simulink model "zad73_dir2slx"  (R2015a)
settings: Solver=FixedStepDiscrete  StartTime=0.0  StopTime=99.0  FixedStep=1  RelTol=1e-3
settings Model: Creator=Bojana Vasic  LastModifiedBy=Bojana Vasic

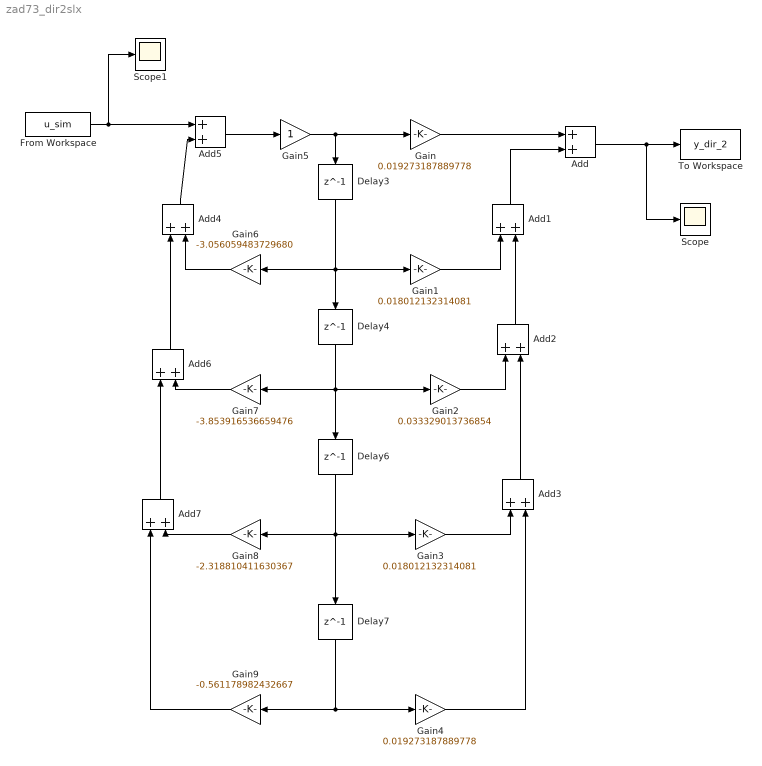
== system zad73_dir2slx ==
  Add{,1..7} (8 alike) : Sum
  Delay{3..4,6..7} (4 alike) : Delay  DelayLength=1
  From Workspace : FromWorkspace  VariableName=u_sim  SampleTime=1
  Gain : Gain  Gain=0.019273187889778
  Gain1 : Gain  Gain=0.018012132314081
  Gain2 : Gain  Gain=0.033329013736854
  Gain3 : Gain  Gain=0.018012132314081
  Gain4 : Gain  Gain=0.019273187889778
  Gain5 : Gain
  Gain6 : Gain  Gain=-3.056059483729680
  Gain7 : Gain  Gain=-3.853916536659476
  Gain8 : Gain  Gain=-2.318810411630367
  Gain9 : Gain  Gain=-0.561178982432667
  Scope : Scope
  Scope1 : Scope
  To Workspace : ToWorkspace  VariableName=y_dir_2  SampleTime=-1
      settings: Save2DSignal=2-D array (concatenate along first dimension)
  wires:
  From Workspace/1 -> Scope1/1, Add5/1
  Add4/1 -> Add5/2
  Gain6/1 -> Add4/2
  Add6/1 -> Add4/1
  Gain7/1 -> Add6/2
  Delay3/1 -> Gain6/1, Gain1/1, Delay4/1
  Add5/1 -> Gain5/1
  Delay4/1 -> Gain2/1, Delay6/1, Gain7/1
  Add7/1 -> Add6/1
  Gain8/1 -> Add7/2
  Delay6/1 -> Gain8/1, Gain3/1, Delay7/1
  Gain9/1 -> Add7/1
  Gain/1 -> Add/1
  Gain1/1 -> Add1/1
  Add1/1 -> Add/2
  Gain2/1 -> Add2/1
  Add2/1 -> Add1/2
  Gain3/1 -> Add3/1
  Add3/1 -> Add2/2
  Delay7/1 -> Gain4/1, Gain9/1
  Gain4/1 -> Add3/2
  Gain5/1 -> Gain/1, Delay3/1
  Add/1 -> Scope/1, To Workspace/1
